simulink model "motor"  (R2024a)
settings: Solver=VariableStepAuto  StartTime=0.0  StopTime=10.0  RelTol=1e-3
libraries: simulink x5, rllib x1
settings Model: Creator=yingb  LastModifiedBy=yingb

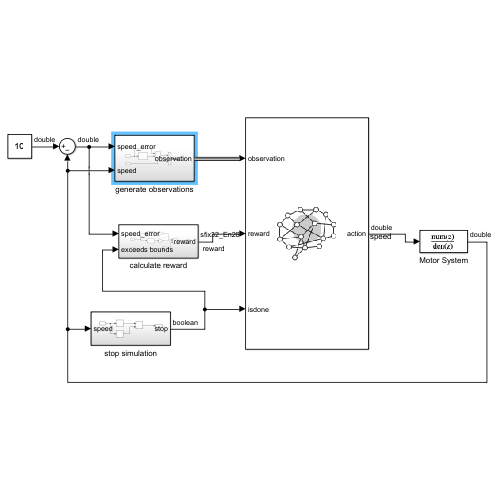
[thumbnail: Simulink's stored preview of the top-level diagram]
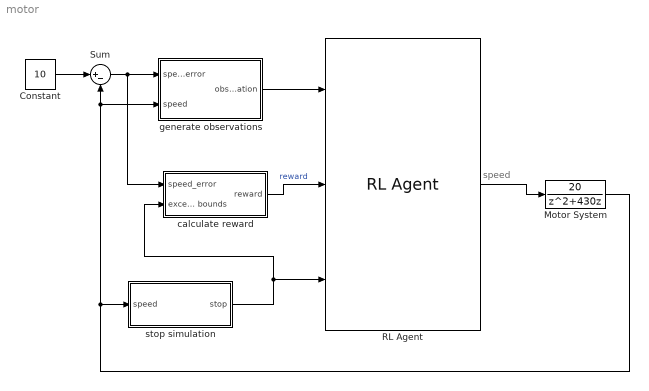
== system motor ==
  note: speed
  Constant : Constant  Value=10
  Motor System : DiscreteTransferFcn  Numerator=20  Denominator=[1 430 0]  StateName=Motor System
  RL Agent : rllib/RL Agent  Agent=agentObj  ExternalActionAsInput=off  ProvideLastAction=off  ProvideCumRwd=off  TreatAsDirectFeedthrough=on  UseStrictObservationDataTypes=off
  Sum : Sum  Inputs=|+-
  calculate reward : Subsystem
  generate observations : Subsystem
  stop simulation : Subsystem
  wires:
  Constant/1 -> Sum/1
  Sum/1 -> calculate reward/1(speed_error), generate observations/1(speed_error)
  calculate reward/1(reward) -> RL Agent/2  "reward"
  stop simulation/1(stop) -> RL Agent/3, calculate reward/2(exceeds bounds)
  RL Agent/1 -> Motor System/1
  Motor System/1 -> stop simulation/1(speed), generate observations/2(speed), Sum/2
  generate observations/1(observation) -> RL Agent/1

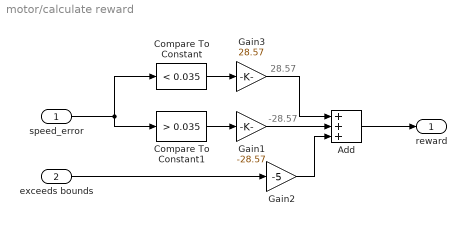
== system motor/calculate reward ==
  note: -28.57
  note: 28.57
  speed_error : Inport
  exceeds bounds : Inport  Port=2
  Add : Sum  Inputs=+++
  Compare To Constant : simulink/Logic and Bit Operations/Compare To Constant  relop=<  const=0.035  OutDataTypeStr=boolean
  Compare To Constant1 : simulink/Logic and Bit Operations/Compare To Constant  relop=>  const=0.035  OutDataTypeStr=boolean
  Gain1 : Gain  Gain=-28.57
  Gain2 : Gain  Gain=-5
  Gain3 : Gain  Gain=28.57
  reward : Outport
  wires:
  exceeds bounds/1 -> Gain2/1
  Gain2/1 -> Add/3
  Add/1 -> reward/1
  speed_error/1 -> Compare To Constant1/1, Compare To Constant/1
  Compare To Constant1/1 -> Gain1/1
  Gain1/1 -> Add/2
  Compare To Constant/1 -> Gain3/1
  Gain3/1 -> Add/1

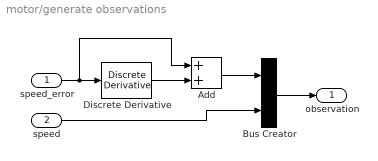
== system motor/generate observations ==
  speed_error : Inport
  speed : Inport  Port=2
  Add : Sum
  Bus Creator : BusCreator  Inputs=2
  Discrete Derivative : simulink/Discrete/Discrete Derivative  gainval=0.05  ICPrevScaledInput=0.0  OutMin=[]  OutMax=[]  OutDataType=fixdt(1, 16)  OutScaling=2^-10  DoSatur=off
  observation : Outport
  wires:
  Discrete Derivative/1 -> Add/2
  speed/1 -> Bus Creator/2
  Add/1 -> Bus Creator/1
  Bus Creator/1 -> observation/1
  speed_error/1 -> Add/1, Discrete Derivative/1

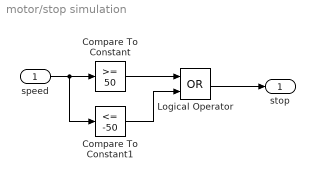
== system motor/stop simulation ==
  speed : Inport
  Compare To Constant : simulink/Logic and Bit Operations/Compare To Constant  relop=>=  const=50  OutDataTypeStr=boolean
  Compare To Constant1 : simulink/Logic and Bit Operations/Compare To Constant  relop=<=  const=-50  OutDataTypeStr=boolean
  Logical Operator : Logic  Operator=OR  AllPortsSameDT=off  OutDataTypeStr=boolean
  stop : Outport
  wires:
  Compare To Constant/1 -> Logical Operator/1
  Compare To Constant1/1 -> Logical Operator/2
  Logical Operator/1 -> stop/1
  speed/1 -> Compare To Constant1/1, Compare To Constant/1
